simulink model "simFile2"  (R2021a)
settings: Solver=FixedStepDiscrete  StartTime=0.0  StopTime=t(end)  FixedStep=TsH  MaxStep=TsH  RelTol=1e-3
values from neighbouring files (symbols this model uses):
  Kd = c2d(K,TsL,'zoh')    [MRStandardPlantLPMExample.m]    (also in SIMOLPMTest.m = c2d(ss(K),Ts))
  Pd = c2d(P,TsH,'zoh')    [MRStandardPlantLPMExample.m]    (also in SIMOLPMTest.m = c2d(P,Ts,'zoh'))
  TsH = 1/fs    (= 0.005)    [MRStandardPlantLPMExample.m]    (also in MultiRateLPM.m; MultiratePFG.m; unliftfrd.m = TsL/F; unliftfrdWithoutRep.m = GliftSIMO.Ts)
  TsL = 1/fsL    (= 0.025)    [MRStandardPlantLPMExample.m]    (also in MultiRateLPM.m = 0.01; MultiratePFG.m = 0.01; unliftfrd.m = GliftSIMO.Ts)
libraries: simulink x1, dspsrcs4 x1
settings Model: Creator=s152009  LastModifiedBy=s152009
settings DebuggingCC: AlgebraicLoopMsg=none

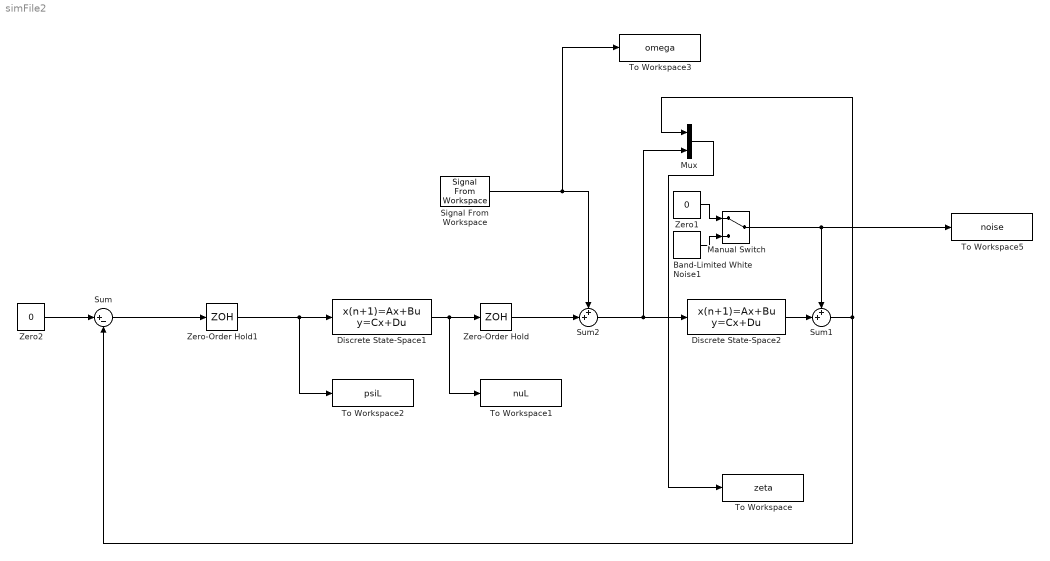
== system simFile2 ==
  Band-Limited White Noise1 : simulink/Sources/Band-Limited White Noise  Cov=0.00000001  Ts=TsH  seed=[23341]
  Discrete State-Space1 : DiscreteStateSpace  A=ss(Kd).A  B=ss(Kd).B  C=ss(Kd).C  D=ss(Kd).D  SampleTime=TsL
  Discrete State-Space2 : DiscreteStateSpace  A=ss(Pd).A  B=ss(Pd).B  C=ss(Pd).C  D=ss(Pd).D  SampleTime=TsH
  Manual Switch : ManualSwitch
  Mux : Mux  Inputs=2
  Signal From Workspace : dspsrcs4/Signal From Workspace  X=rHexp  Ts=TsH  nsamps=1  OutputAfterFinalValue=Setting to zero  ignoreOrWarnInputAndFrameLengths=off  OutputFrames=off
  Sum : Sum  Inputs=|+-
  Sum1 : Sum  Inputs=++|
  Sum2 : Sum  Inputs=++|
  To Workspace : ToWorkspace  VariableName=zeta  SampleTime=TsH
      settings: Save2DSignal=2-D array (concatenate along first dimension)
  To Workspace1 : ToWorkspace  VariableName=nuL  SampleTime=TsL
      settings: Save2DSignal=2-D array (concatenate along first dimension)
  To Workspace2 : ToWorkspace  VariableName=psiL  SampleTime=TsL
      settings: Save2DSignal=2-D array (concatenate along first dimension)
  To Workspace3 : ToWorkspace  VariableName=omega  SampleTime=TsH
      settings: Save2DSignal=2-D array (concatenate along first dimension)
  To Workspace5 : ToWorkspace  VariableName=noise  SampleTime=TsH
      settings: Save2DSignal=2-D array (concatenate along first dimension)
  Zero-Order Hold : ZeroOrderHold  SampleTime=TsH
  Zero-Order Hold1 : ZeroOrderHold  SampleTime=TsL
  Zero1 : Constant  Value=0  OutDataTypeStr=Inherit: Inherit via back propagation
  Zero2 : Constant  Value=0  OutDataTypeStr=Inherit: Inherit via back propagation
  wires:
  Sum/1 -> Zero-Order Hold1/1
  Zero-Order Hold1/1 -> To Workspace2/1, Discrete State-Space1/1
  Discrete State-Space1/1 -> To Workspace1/1, Zero-Order Hold/1
  Mux/1 -> To Workspace/1
  Band-Limited White Noise1/1 -> Manual Switch/2
  Zero1/1 -> Manual Switch/1
  Discrete State-Space2/1 -> Sum1/2
  Sum1/1 -> Mux/1, Sum/2
  Manual Switch/1 -> To Workspace5/1, Sum1/1
  Zero-Order Hold/1 -> Sum2/2
  Sum2/1 -> Mux/2, Discrete State-Space2/1
  Zero2/1 -> Sum/1
  Signal From Workspace/1 -> Sum2/1, To Workspace3/1
